simulink library "DYN"  (Simulink 10.1)
settings: Solver=VariableStepAuto  StartTime=0.0  StopTime=10.0  RelTol=1e-3
undefined symbols (not defined in the file): DYN_MAG_par, DYN_SC_par
libraries: DYN_AERO x1, DYN_ATT x1, DYN_EPHEM x1, DYN_GRAV x1, DYN_MAG x1, DYN_TIME x1, DYN_TRA x1
settings Model: Creator=WilTravis  LastModifiedBy=m_mam

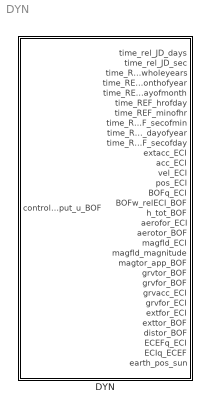
== system DYN ==
  DYN : Subsystem

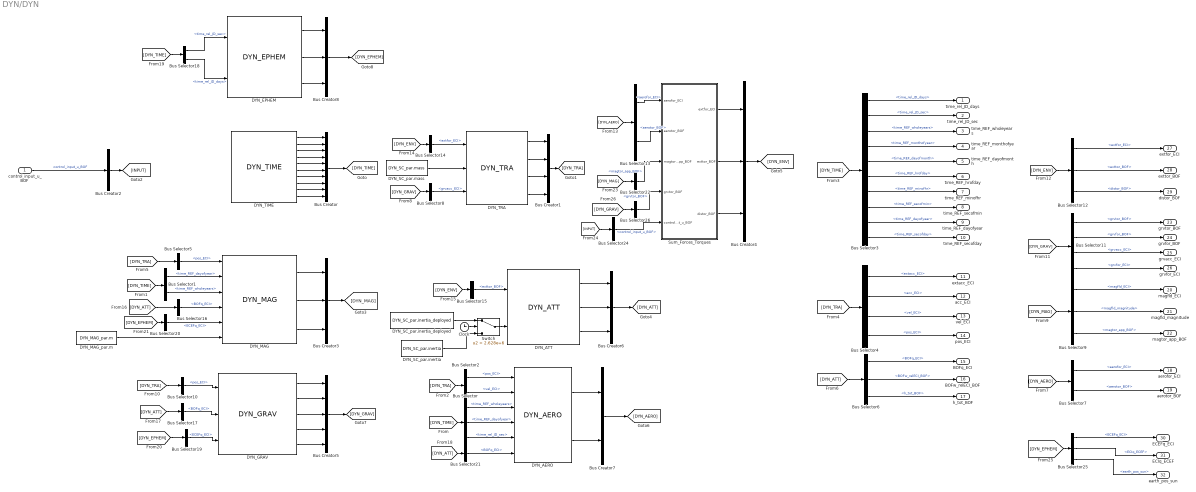
== system DYN/DYN ==
  control_input_u_BOF : Inport
  Bus Creator : BusCreator  Inputs=10
  Bus Creator1 : BusCreator  Inputs=4
  Bus Creator2 : BusCreator  Inputs=1
  Bus Creator{3..4,6,8} (4 alike) : BusCreator  Inputs=3
  Bus Creator5 : BusCreator  Inputs=5
  Bus Creator7 : BusCreator  Inputs=2
  Bus Selector : BusSelector  OutputSignals=time_REF_wholeyears,time_REF_dayofyear,time_rel_JD_sec
  Bus Selector1 : BusSelector  OutputSignals=time_REF_dayofyear,time_REF_wholeyears
  Bus Selector10 : BusSelector  OutputSignals=pos_ECI
  Bus Selector11 : BusSelector  OutputSignals=grvtor_BOF,grvfor_BOF,grvacc_ECI,grvfor_ECI
  Bus Selector12 : BusSelector  OutputSignals=extfor_ECI,exttor_BOF,distor_BOF
  Bus Selector13 : BusSelector  OutputSignals=aerofor_ECI,aerotor_BOF
  Bus Selector14 : BusSelector  OutputSignals=extfor_ECI
  Bus Selector15 : BusSelector  OutputSignals=exttor_BOF
  Bus Selector16 : BusSelector  OutputSignals=BOFq_ECI
  Bus Selector17 : BusSelector  OutputSignals=BOFq_ECI
  Bus Selector18 : BusSelector  OutputSignals=time_rel_JD_sec,time_rel_JD_days
  Bus Selector19 : BusSelector  OutputSignals=ECEFq_ECI
  Bus Selector2 : BusSelector  OutputSignals=pos_ECI,vel_ECI
  Bus Selector20 : BusSelector  OutputSignals=ECEFq_ECI
  Bus Selector21 : BusSelector  OutputSignals=BOFq_ECI
  Bus Selector22 : BusSelector  OutputSignals=magtor_app_BOF
  Bus Selector24 : BusSelector  OutputSignals=control_input_u_BOF
  Bus Selector25 : BusSelector  OutputSignals=ECEFq_ECI,ECIq_ECEF,earth_pos_sun
  Bus Selector26 : BusSelector  OutputSignals=grvtor_BOF
  Bus Selector3 : BusSelector  OutputSignals=time_rel_JD_days,time_rel_JD_sec,time_REF_wholeyears,time_REF_monthofyear,time_REF_dayofmonth,time_REF_hrofday,time_REF_minofhr,time_REF_secofmin,time_REF_dayofyear,time_REF_secofday
  Bus Selector4 : BusSelector  OutputSignals=extacc_ECI,acc_ECI,vel_ECI,pos_ECI
  Bus Selector5 : BusSelector  OutputSignals=pos_ECI
  Bus Selector6 : BusSelector  OutputSignals=BOFq_ECI,BOFw_relECI_BOF,h_tot_BOF
  Bus Selector7 : BusSelector  OutputSignals=aerofor_ECI,aerotor_BOF
  Bus Selector8 : BusSelector  OutputSignals=grvacc_ECI
  Bus Selector9 : BusSelector  OutputSignals=magfld_ECI,magfld_magnitude,magtor_app_BOF
  Clock : Clock
  DYN_AERO : DYN_AERO/DYN_AERO  SystemSampleTime=-1  Latency=0  AutoFrameSizeCalculation=off
  DYN_ATT : DYN_ATT/DYN_ATT  SystemSampleTime=-1  Latency=0  AutoFrameSizeCalculation=off
  DYN_EPHEM : DYN_EPHEM/DYN_EPHEM  SystemSampleTime=-1  Latency=0  AutoFrameSizeCalculation=off
  DYN_GRAV : DYN_GRAV/DYN_GRAV  SystemSampleTime=-1  Latency=0  AutoFrameSizeCalculation=off
  DYN_MAG : DYN_MAG/DYN_MAG  SystemSampleTime=-1  Latency=0  AutoFrameSizeCalculation=off
  DYN_MAG_par.m : Constant  Value=DYN_MAG_par.m
  DYN_SC_par.inertia : Constant  Value=DYN_SC_par.inertia
  DYN_SC_par.inertia_deployed : Constant  Value=DYN_SC_par.inertia_deployed
  DYN_SC_par.mass : Constant  Value=DYN_SC_par.mass
  DYN_TIME : DYN_TIME/DYN_TIME  SystemSampleTime=-1  Latency=0  AutoFrameSizeCalculation=off
  DYN_TRA : DYN_TRA/DYN_TRA  SystemSampleTime=-1  Latency=0  AutoFrameSizeCalculation=off
  Sum_Forces_Torques : Subsystem
  Switch : Switch  Criteria=u2 > Threshold  Threshold=2.628e+6
  time_rel_JD_days : Outport  VectorParamsAs1DForOutWhenUnconnected=off
  time_rel_JD_sec : Outport  Port=2  VectorParamsAs1DForOutWhenUnconnected=off
  time_REF_wholeyears : Outport  Port=3  VectorParamsAs1DForOutWhenUnconnected=off
  time_REF_monthofyear : Outport  Port=4  VectorParamsAs1DForOutWhenUnconnected=off
  time_REF_dayofmonth : Outport  Port=5  VectorParamsAs1DForOutWhenUnconnected=off
  time_REF_hrofday : Outport  Port=6  VectorParamsAs1DForOutWhenUnconnected=off
  time_REF_minofhr : Outport  Port=7  VectorParamsAs1DForOutWhenUnconnected=off
  time_REF_secofmin : Outport  Port=8  VectorParamsAs1DForOutWhenUnconnected=off
  time_REF_dayofyear : Outport  Port=9  VectorParamsAs1DForOutWhenUnconnected=off
  time_REF_secofday : Outport  Port=10  VectorParamsAs1DForOutWhenUnconnected=off
  extacc_ECI : Outport  Port=11  VectorParamsAs1DForOutWhenUnconnected=off
  acc_ECI : Outport  Port=12  VectorParamsAs1DForOutWhenUnconnected=off
  vel_ECI : Outport  Port=13  VectorParamsAs1DForOutWhenUnconnected=off
  pos_ECI : Outport  Port=14  VectorParamsAs1DForOutWhenUnconnected=off
  "BOFq_ECI " : Outport  Port=15  VectorParamsAs1DForOutWhenUnconnected=off
  "BOFw_relECI_BOF " : Outport  Port=16  VectorParamsAs1DForOutWhenUnconnected=off
  h_tot_BOF : Outport  Port=17  VectorParamsAs1DForOutWhenUnconnected=off
  aerofor_ECI : Outport  Port=18  VectorParamsAs1DForOutWhenUnconnected=off
  aerotor_BOF : Outport  Port=19  VectorParamsAs1DForOutWhenUnconnected=off
  magfld_ECI : Outport  Port=20  VectorParamsAs1DForOutWhenUnconnected=off
  magfld_magnitude : Outport  Port=21  VectorParamsAs1DForOutWhenUnconnected=off
  "magtor_app_BOF " : Outport  Port=22  VectorParamsAs1DForOutWhenUnconnected=off
  "grvtor_BOF " : Outport  Port=23  VectorParamsAs1DForOutWhenUnconnected=off
  "grvfor_BOF " : Outport  Port=24  VectorParamsAs1DForOutWhenUnconnected=off
  grvacc_ECI : Outport  Port=25  VectorParamsAs1DForOutWhenUnconnected=off
  grvfor_ECI : Outport  Port=26  VectorParamsAs1DForOutWhenUnconnected=off
  extfor_ECI : Outport  Port=27  VectorParamsAs1DForOutWhenUnconnected=off
  exttor_BOF : Outport  Port=28  VectorParamsAs1DForOutWhenUnconnected=off
  distor_BOF : Outport  Port=29  VectorParamsAs1DForOutWhenUnconnected=off
  ECEFq_ECI : Outport  Port=30  VectorParamsAs1DForOutWhenUnconnected=off
  ECIq_ECEF : Outport  Port=31  VectorParamsAs1DForOutWhenUnconnected=off
  earth_pos_sun : Outport  Port=32  VectorParamsAs1DForOutWhenUnconnected=off
  wires:
  Bus Selector25/3 -> earth_pos_sun/1  "<earth_pos_sun>"
  DYN_EPHEM/3 -> Bus Creator8/3
  Bus Selector18/2 -> DYN_EPHEM/2  "<time_rel_JD_days>"
  [DYN_TIME] -> Bus Selector/1
  [DYN_TIME] -> Bus Selector1/1
  Bus Creator1/1 -> [DYN_TRA]
  [DYN_TRA] -> Bus Selector2/1
  [DYN_TIME] -> Bus Selector3/1
  Bus Selector3/1 -> time_rel_JD_days/1  "<time_rel_JD_days>"
  Bus Selector3/2 -> time_rel_JD_sec/1  "<time_rel_JD_sec>"
  Bus Selector3/3 -> time_REF_wholeyears/1  "<time_REF_wholeyears>"
  Bus Selector3/4 -> time_REF_monthofyear/1  "<time_REF_monthofyear>"
  Bus Selector3/5 -> time_REF_dayofmonth/1  "<time_REF_dayofmonth>"
  Bus Selector3/6 -> time_REF_hrofday/1  "<time_REF_hrofday>"
  Bus Selector3/7 -> time_REF_minofhr/1  "<time_REF_minofhr>"
  Bus Selector3/8 -> time_REF_secofmin/1  "<time_REF_secofmin>"
  Bus Selector3/9 -> time_REF_dayofyear/1  "<time_REF_dayofyear>"
  Bus Selector3/10 -> time_REF_secofday/1  "<time_REF_secofday>"
  DYN_TIME/1 -> Bus Creator/1
  DYN_TIME/2 -> Bus Creator/2
  DYN_TIME/3 -> Bus Creator/3
  DYN_TIME/4 -> Bus Creator/4
  DYN_TIME/5 -> Bus Creator/5
  DYN_TIME/6 -> Bus Creator/6
  DYN_TIME/7 -> Bus Creator/7
  DYN_TIME/8 -> Bus Creator/8
  DYN_TIME/9 -> Bus Creator/9
  DYN_TIME/10 -> Bus Creator/10
  Bus Creator/1 -> [DYN_TIME]
  [DYN_TRA] -> Bus Selector4/1
  Bus Selector4/1 -> extacc_ECI/1  "<extacc_ECI>"
  Bus Selector4/2 -> acc_ECI/1  "<acc_ECI>"
  Bus Selector4/3 -> vel_ECI/1  "<vel_ECI>"
  Bus Selector4/4 -> pos_ECI/1  "<pos_ECI>"
  Bus Creator2/1 -> [INPUT]
  Bus Creator3/1 -> [DYN_MAG]
  [DYN_TRA] -> Bus Selector5/1
  Bus Selector5/1 -> DYN_MAG/1  "<pos_ECI>"
  DYN_SC_par.mass/1 -> DYN_TRA/2
  [DYN_GRAV] -> Bus Selector8/1
  Bus Creator4/1 -> [DYN_ENV]
  Sum_Forces_Torques/1(extfor_ECI) -> Bus Creator4/1
  [DYN_TRA] -> Bus Selector10/1
  Bus Selector10/1 -> DYN_GRAV/1  "<pos_ECI>"
  Bus Creator5/1 -> [DYN_GRAV]
  DYN_GRAV/1 -> Bus Creator5/1
  DYN_GRAV/2 -> Bus Creator5/2
  DYN_GRAV/3 -> Bus Creator5/3
  Bus Selector8/1 -> DYN_TRA/3  "<grvacc_ECI>"
  DYN_TRA/4 -> Bus Creator1/4
  DYN_TRA/3 -> Bus Creator1/3
  DYN_TRA/2 -> Bus Creator1/2
  DYN_TRA/1 -> Bus Creator1/1
  DYN_MAG/1 -> Bus Creator3/1
  DYN_MAG/3 -> Bus Creator3/3
  DYN_MAG/2 -> Bus Creator3/2
  Bus Selector2/1 -> DYN_AERO/1  "<pos_ECI>"
  DYN_ATT/2 -> Bus Creator6/2
  DYN_ATT/3 -> Bus Creator6/3
  DYN_ATT/1 -> Bus Creator6/1
  Bus Creator6/1 -> [DYN_ATT]
  DYN_AERO/1 -> Bus Creator7/1
  DYN_AERO/2 -> Bus Creator7/2
  Bus Creator7/1 -> [DYN_AERO]
  [DYN_ATT] -> Bus Selector6/1
  Bus Selector6/1 -> "BOFq_ECI "/1  "<BOFq_ECI>"
  Bus Selector6/2 -> "BOFw_relECI_BOF "/1  "<BOFw_relECI_BOF>"
  Bus Selector6/3 -> h_tot_BOF/1  "<h_tot_BOF>"
  [DYN_AERO] -> Bus Selector7/1
  Bus Selector7/1 -> aerofor_ECI/1  "<aerofor_ECI>"
  Bus Selector7/2 -> aerotor_BOF/1  "<aerotor_BOF>"
  [DYN_MAG] -> Bus Selector9/1
  Bus Selector9/1 -> magfld_ECI/1  "<magfld_ECI>"
  Bus Selector9/2 -> magfld_magnitude/1  "<magfld_magnitude>"
  [DYN_GRAV] -> Bus Selector11/1
  Bus Selector11/3 -> grvacc_ECI/1  "<grvacc_ECI>"
  Bus Selector11/1 -> "grvtor_BOF "/1  "<grvtor_BOF>"
  Bus Selector11/2 -> "grvfor_BOF "/1  "<grvfor_BOF>"
  Bus Selector12/1 -> extfor_ECI/1  "<extfor_ECI>"
  [DYN_ENV] -> Bus Selector12/1
  [DYN_AERO] -> Bus Selector13/1
  Bus Selector13/1 -> Sum_Forces_Torques/1(aerofor_ECI)  "<aerofor_ECI>"
  Bus Selector13/2 -> Sum_Forces_Torques/2(aerotor_BOF)  "<aerotor_BOF>"
  [DYN_ENV] -> Bus Selector14/1
  Bus Selector14/1 -> DYN_TRA/1  "<extfor_ECI>"
  [DYN_ENV] -> Bus Selector15/1
  Bus Selector15/1 -> DYN_ATT/1  "<exttor_BOF>"
  [DYN_ATT] -> Bus Selector16/1
  Bus Selector17/1 -> DYN_GRAV/2  "<BOFq_ECI>"
  [DYN_ATT] -> Bus Selector17/1
  [DYN_TIME] -> Bus Selector18/1
  Bus Selector18/1 -> DYN_EPHEM/1  "<time_rel_JD_sec>"
  DYN_EPHEM/1 -> Bus Creator8/1
  DYN_EPHEM/2 -> Bus Creator8/2
  Bus Creator8/1 -> [DYN_EPHEM]
  [DYN_EPHEM] -> Bus Selector19/1
  Bus Selector19/1 -> DYN_GRAV/3  "<ECEFq_ECI>"
  [DYN_EPHEM] -> Bus Selector20/1
  DYN_GRAV/4 -> Bus Creator5/4
  [DYN_MAG] -> Bus Selector22/1
  Bus Selector22/1 -> Sum_Forces_Torques/3(magtor_app_BOF)  "<magtor_app_BOF>"
  Bus Selector1/1 -> DYN_MAG/2  "<time_REF_dayofyear>"
  Bus Selector16/1 -> DYN_MAG/4  "<BOFq_ECI>"
  DYN_MAG_par.m/1 -> DYN_MAG/6
  [DYN_ATT] -> Bus Selector21/1
  Bus Selector21/1 -> DYN_AERO/6  "<BOFq_ECI>"
  Sum_Forces_Torques/2(exttor_BOF) -> Bus Creator4/2
  Bus Selector12/2 -> exttor_BOF/1  "<exttor_BOF>"
  [DYN_EPHEM] -> Bus Selector25/1
  Bus Selector25/1 -> ECEFq_ECI/1  "<ECEFq_ECI>"
  Bus Selector25/2 -> ECIq_ECEF/1  "<ECIq_ECEF>"
  [DYN_GRAV] -> Bus Selector26/1
  Bus Selector26/1 -> Sum_Forces_Torques/4(grvtor_BOF)  "<grvtor_BOF>"
  Bus Selector1/2 -> DYN_MAG/3  "<time_REF_wholeyears>"
  Bus Selector20/1 -> DYN_MAG/5  "<ECEFq_ECI>"
  Bus Selector2/2 -> DYN_AERO/2  "<vel_ECI>"
  Bus Selector/1 -> DYN_AERO/3  "<time_REF_wholeyears>"
  Bus Selector/2 -> DYN_AERO/4  "<time_REF_dayofyear>"
  Bus Selector/3 -> DYN_AERO/5  "<time_rel_JD_sec>"
  DYN_GRAV/5 -> Bus Creator5/5
  Bus Selector11/4 -> grvfor_ECI/1  "<grvfor_ECI>"
  Bus Selector9/3 -> "magtor_app_BOF "/1  "<magtor_app_BOF>"
  control_input_u_BOF/1 -> Bus Creator2/1  "control_input_u_BOF"
  [INPUT] -> Bus Selector24/1
  Bus Selector24/1 -> Sum_Forces_Torques/5(control_input_u_BOF)  "<control_input_u_BOF>"
  DYN_SC_par.inertia/1 -> Switch/3
  Switch/1 -> DYN_ATT/2
  DYN_SC_par.inertia_deployed/1 -> Switch/1
  Clock/1 -> Switch/2
  Sum_Forces_Torques/3(distor_BOF) -> Bus Creator4/3
  Bus Selector12/3 -> distor_BOF/1  "<distor_BOF>"

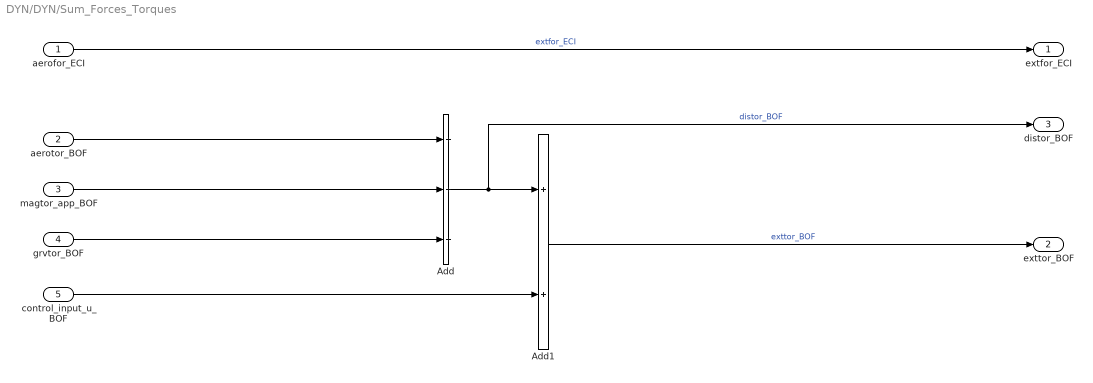
== system DYN/DYN/Sum_Forces_Torques ==
  aerofor_ECI : Inport
  aerotor_BOF : Inport  Port=2
  magtor_app_BOF : Inport  Port=3
  grvtor_BOF : Inport  Port=4
  control_input_u_BOF : Inport  Port=5
  Add : Sum  Inputs=+++
  Add1 : Sum
  extfor_ECI : Outport  VectorParamsAs1DForOutWhenUnconnected=off
  exttor_BOF : Outport  Port=2  VectorParamsAs1DForOutWhenUnconnected=off
  distor_BOF : Outport  Port=3  VectorParamsAs1DForOutWhenUnconnected=off
  wires:
  Add1/1 -> exttor_BOF/1  "exttor_BOF"
  aerofor_ECI/1 -> extfor_ECI/1  "extfor_ECI"
  Add/1 -> distor_BOF/1, Add1/1  "distor_BOF"
  aerotor_BOF/1 -> Add/1
  magtor_app_BOF/1 -> Add/2
  grvtor_BOF/1 -> Add/3
  control_input_u_BOF/1 -> Add1/2
